simulink model "HexWaRo_StAc_WS_MD"  (Simulink 8.0)
settings: Solver=ode3  StartTime=0.0  StopTime=SimTime  FixedStep=0.02  RelTol=1e-3
values from neighbouring files (symbols this model uses):
  Dgain = -50    [ContinLearn.m]    (also in LearnEvaluation.m; StAcEval.m)
  Kgain = -1500    [ContinLearn.m]    (also in LearnEvaluation.m; StAcEval.m)
  SimTime = .5    (= 0.5)    [ContinLearn.m]    (also in LearnEvaluation.m; StAcEval.m)
  ThetaB = StDeg(st)    [ContinLearn.m]    (also in LearnEvaluation.m; StAcEval.m)
  ThetaE = StDeg(ac)    [ContinLearn.m]    (also in LearnEvaluation.m; StAcEval.m)
libraries: mblibv1 x86
(part 2 of 2)

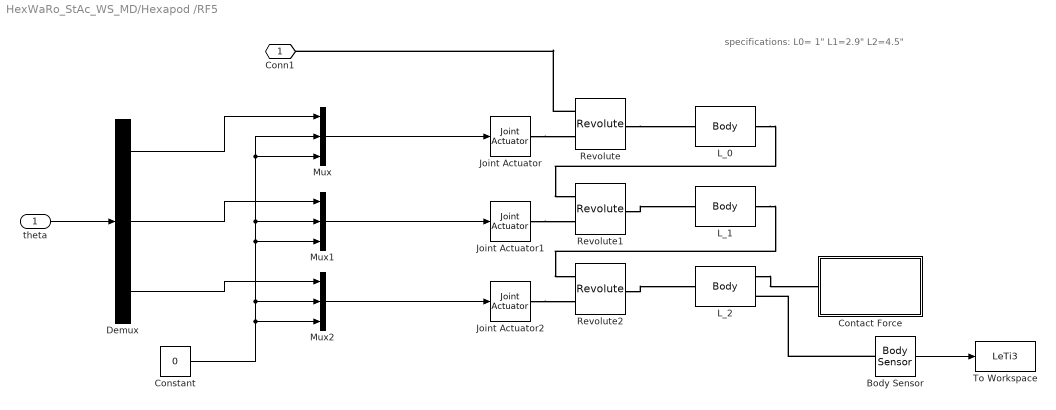
== system HexWaRo_StAc_WS_MD/Hexapod /RF5 ==
  note: specifications:
      | L0= 1"
      | L1=2.9"
      | L2=4.5"
  "theta " : Inport
  Body Sensor : mblibv1/Sensors &  Actuators/Body Sensor  UpdateFromCAD=off  PhysicalDomain=Mechanical  PortType=blob  Muxed=on  Pose=off  Angle=on  AngleUnits=deg  ArcVelocity=off  ArcVelocityUnits=deg/s  ArcAcceleration=off  ArcAccelerationUnits=deg/s^2  CoordPosition=on  CoordPositionUnits=m  Velocity=off  VelocityUnits=m/s  Acceleration=off  AccelerationUnits=m/s^2  Quaternion=on  QuaternionDT=off  QuaternionDDT=off  QuaternionUnits=off  OutputVector=[1]  ActiveIO=on  Width=3  DialogClass=MechanicalSensorBlock  ReferenceFrame=Absolute (World)
  Constant : Constant  Value=0
  Contact Force : Subsystem
  Demux : Demux  Outputs=3
  Joint Actuator : mblibv1/Sensors &  Actuators/Joint Actuator  UpdateFromCAD=off  PhysicalDomain=Mechanical  PortType=blob  ActuationStyle=Motion  AngleUnits=rad  ArcVelocityUnits=rad/s  ArcAccelerationUnits=deg/s^2  CoordPositionUnits=m  VelocityUnits=m/s  AccelerationUnits=m/s^2  ForceUnits=N  TorqueUnits=N*m  ActiveIO=on  Width=3  DialogClass=MechanicalActuatorBlock  Primitive=R1  ReferenceFrame=Absolute (World)
  Joint Actuator1 : mblibv1/Sensors &  Actuators/Joint Actuator  UpdateFromCAD=off  PhysicalDomain=Mechanical  PortType=blob  ActuationStyle=Motion  AngleUnits=rad  ArcVelocityUnits=deg/s  ArcAccelerationUnits=deg/s^2  CoordPositionUnits=m  VelocityUnits=m/s  AccelerationUnits=m/s^2  ForceUnits=N  TorqueUnits=N*m  ActiveIO=on  Width=3  DialogClass=MechanicalActuatorBlock  Primitive=R1  ReferenceFrame=Absolute (World)
  Joint Actuator2 : mblibv1/Sensors &  Actuators/Joint Actuator  UpdateFromCAD=off  PhysicalDomain=Mechanical  PortType=blob  ActuationStyle=Motion  AngleUnits=rad  ArcVelocityUnits=deg/s  ArcAccelerationUnits=deg/s^2  CoordPositionUnits=m  VelocityUnits=m/s  AccelerationUnits=m/s^2  ForceUnits=N  TorqueUnits=N*m  ActiveIO=on  Width=3  DialogClass=MechanicalActuatorBlock  Primitive=R1  ReferenceFrame=Absolute (World)
  L_0 : mblibv1/Bodies/Body  LConnTagsString=CS1  RConnTagsString=CS2  UpdateFromCAD=off  DialogClass=MechanicalBodyBlock  Mass=.1  MassUnits=kg  InertiaUnits=kg*m^2  Inertia=eye(3)  Shape=Cylinder  ShapeDims=[1 1]  ShapeUnits=m  ShapeUse=false  Density=1  DensityUnits=kg/m^3  DensityUse=false  GraphicsMode=MACHINE_DEFAULT  BodyColorSelMode=MACHINE_DEFAULT  BodyColor=[1 0 0]  AttachedToCS=CG  CG=Left$CG$[1.25 0 0]$CS1$CS1$cm$[0 0 0]$Euler X-Y-Z$deg$WORLD$false$none  WorkingFrames=Left$CS1$[0 0 0]$Adjoining$Adjoining$cm$[0 0 0]$Euler X-Y-Z$deg$WORLD$true$none#Right$CS2$[2.5 0 0]$CS1$CS1$cm$[0 0 0]$Euler X-Y-Z$deg$WORLD$true$none  CGPos=[1.25 0 0]  CGRot=[0 0 0]  CS0Pos=[]  CS0Rot=[]  CS1Pos=[0 0 0]  CS1Rot=[0 0 0]  CS2Pos=[2.5 0 0]  CS2Rot=[0 0 0]  CS3Pos=[]  CS3Rot=[]  CS4Pos=[]  CS4Rot=[]  CS5Pos=[]  CS5Rot=[]  CS6Pos=[]  CS6Rot=[]  CS7Pos=[]  CS7Rot=[]  CS8Pos=[]  CS8Rot=[]  CS9Pos=[]  CS9Rot=[]  CS10Pos=[]  CS10Rot=[]  CS11Pos=[]  CS11Rot=[]  CS12Pos=[]  CS12Rot=[]  CS13Pos=[]  CS13Rot=[]  CS14Pos=[]  CS14Rot=[]  CS15Pos=[]  CS15Rot=[]  CS16Pos=[]  CS16Rot=[]  CS17Pos=[]  CS17Rot=[]  CS18Pos=[]  CS18Rot=[]  CS19Pos=[]  CS19Rot=[]  CS20Pos=[]  CS20Rot=[]
  L_1 : mblibv1/Bodies/Body  LConnTagsString=CS1  RConnTagsString=CS2  UpdateFromCAD=off  DialogClass=MechanicalBodyBlock  Mass=.1  MassUnits=kg  InertiaUnits=kg*m^2  Inertia=eye(3)  Shape=Cylinder  ShapeDims=[1 1]  ShapeUnits=m  ShapeUse=false  Density=1  DensityUnits=kg/m^3  DensityUse=false  GraphicsMode=MACHINE_DEFAULT  BodyColorSelMode=MACHINE_DEFAULT  BodyColor=[1 0 0]  AttachedToCS=CG  CG=Left$CG$[3.7 0 0]$CS1$CS1$cm$[0 0 0]$Euler X-Y-Z$deg$WORLD$false$none  WorkingFrames=Left$CS1$[0 0 0]$Adjoining$Adjoining$cm$[0 0 0]$Euler X-Y-Z$deg$WORLD$true$none#Right$CS2$[7.4 0 0]$CS1$CS1$cm$[0 0 0]$Euler X-Y-Z$deg$WORLD$true$none  CGPos=[3.7 0 0]  CGRot=[0 0 0]  CS0Pos=[]  CS0Rot=[]  CS1Pos=[0 0 0]  CS1Rot=[0 0 0]  CS2Pos=[7.4 0 0]  CS2Rot=[0 0 0]  CS3Pos=[]  CS3Rot=[]  CS4Pos=[]  CS4Rot=[]  CS5Pos=[]  CS5Rot=[]  CS6Pos=[]  CS6Rot=[]  CS7Pos=[]  CS7Rot=[]  CS8Pos=[]  CS8Rot=[]  CS9Pos=[]  CS9Rot=[]  CS10Pos=[]  CS10Rot=[]  CS11Pos=[]  CS11Rot=[]  CS12Pos=[]  CS12Rot=[]  CS13Pos=[]  CS13Rot=[]  CS14Pos=[]  CS14Rot=[]  CS15Pos=[]  CS15Rot=[]  CS16Pos=[]  CS16Rot=[]  CS17Pos=[]  CS17Rot=[]  CS18Pos=[]  CS18Rot=[]  CS19Pos=[]  CS19Rot=[]  CS20Pos=[]  CS20Rot=[]
  L_2 : mblibv1/Bodies/Body  LConnTagsString=CS1  RConnTagsString=CS2|CS3  UpdateFromCAD=off  DialogClass=MechanicalBodyBlock  Mass=.1  MassUnits=kg  InertiaUnits=kg*m^2  Inertia=eye(3)  Shape=Cylinder  ShapeDims=[1 1]  ShapeUnits=m  ShapeUse=false  Density=1  DensityUnits=kg/m^3  DensityUse=false  GraphicsMode=MACHINE_DEFAULT  BodyColorSelMode=MACHINE_DEFAULT  BodyColor=[1 0 0]  AttachedToCS=CG  CG=Left$CG$[5.7 0 0]$CS1$CS1$cm$[0 0 0]$Euler X-Y-Z$deg$WORLD$false$none  WorkingFrames=Left$CS1$[0 0 0]$Adjoining$Adjoining$cm$[0 0 0]$Euler X-Y-Z$deg$WORLD$true$none#Right$CS2$[11.4 0 0]$CS1$CS1$cm$[0 0 0]$Euler X-Y-Z$deg$WORLD$true$none#Right$CS3$[11.4 0 0]$CS1$CS1$cm$[0 0 0]$Euler X-Y-Z$deg$WORLD$true$none  CGPos=[5.7 0 0]  CGRot=[0 0 0]  CS0Pos=[]  CS0Rot=[]  CS1Pos=[0 0 0]  CS1Rot=[0 0 0]  CS2Pos=[11.4 0 0]  CS2Rot=[0 0 0]  CS3Pos=[11.4 0 0]  CS3Rot=[0 0 0]  CS4Pos=[]  CS4Rot=[]  CS5Pos=[]  CS5Rot=[]  CS6Pos=[]  CS6Rot=[]  CS7Pos=[]  CS7Rot=[]  CS8Pos=[]  CS8Rot=[]  CS9Pos=[]  CS9Rot=[]  CS10Pos=[]  CS10Rot=[]  CS11Pos=[]  CS11Rot=[]  CS12Pos=[]  CS12Rot=[]  CS13Pos=[]  CS13Rot=[]  CS14Pos=[]  CS14Rot=[]  CS15Pos=[]  CS15Rot=[]  CS16Pos=[]  CS16Rot=[]  CS17Pos=[]  CS17Rot=[]  CS18Pos=[]  CS18Rot=[]  CS19Pos=[]  CS19Rot=[]  CS20Pos=[]  CS20Rot=[]
  Mux : Mux  Inputs=3
  Mux1 : Mux  Inputs=3
  Mux2 : Mux  Inputs=3
  Revolute : mblibv1/Joints/Revolute  LConnTagsString=__newl0|SA1  RConnTagsString=__newr0  UpdateFromCAD=off  NumSAPorts=1  CutJoint=off  MarkAsCut=off  Primitives=prismatic  PrimitiveProps=R1$World$[0 0 1]$revolute  DialogClass=JointBlock  R1Axis=[0 0 1]
  Revolute1 : mblibv1/Joints/Revolute  LConnTagsString=__newl0|SA1  RConnTagsString=__newr0  UpdateFromCAD=off  NumSAPorts=1  CutJoint=off  MarkAsCut=off  Primitives=prismatic  PrimitiveProps=R1$Base$[0 1 0]$revolute  DialogClass=JointBlock  R1Axis=[0 1 0]
  Revolute2 : mblibv1/Joints/Revolute  LConnTagsString=__newl0|SA1  RConnTagsString=__newr0  UpdateFromCAD=off  NumSAPorts=1  CutJoint=off  MarkAsCut=off  Primitives=prismatic  PrimitiveProps=R1$Base$[0 1 0]$revolute  DialogClass=JointBlock  R1Axis=[0 1 0]
  To Workspace : ToWorkspace  VariableName=LeTi3  SampleTime=-1
  Conn1 : PMIOPort  Port=1  Side=Left
  wires:
  "theta "/1 -> Demux/1
  Constant/1 -> Mux2/2, Mux1/3, Mux1/2, Mux/3, Mux/2, Mux2/3
  Demux/3 -> Mux2/1
  Demux/2 -> Mux1/1
  Demux/1 -> Mux/1
  Mux/1 -> Joint Actuator/1
  Mux1/1 -> Joint Actuator1/1
  Mux2/1 -> Joint Actuator2/1
  Body Sensor/1 -> To Workspace/1
  connections:
  Revolute1/RConn1 -- L_1/LConn1
  Revolute2/RConn1 -- L_2/LConn1
  Joint Actuator2/RConn1 -- Revolute2/LConn2
  Joint Actuator/RConn1 -- Revolute/LConn2
  Joint Actuator1/RConn1 -- Revolute1/LConn2
  Revolute/LConn1 -- Conn1/RConn1
  Revolute/RConn1 -- L_0/LConn1
  L_1/RConn1 -- Revolute2/LConn1
  L_0/RConn1 -- Revolute1/LConn1
  L_2/RConn1 -- Contact Force/LConn1
  Body Sensor/LConn1 -- L_2/RConn2

== system HexWaRo_StAc_WS_MD/Hexapod /RF/Contact Force ==
  Body Actuator : mblibv1/Sensors &  Actuators/Body Actuator  UpdateFromCAD=off  PhysicalDomain=Mechanical  PortType=blob  ActuationStyle=Force  AngleUnits=deg  ArcVelocityUnits=deg/s  ArcAccelerationUnits=deg/s^2  CoordPositionUnits=m  VelocityUnits=m/s  AccelerationUnits=m/s^2  ForceUnits=N  TorqueUnits=N-m  ActiveIO=on  Width=3  DialogClass=MechanicalActuatorBlock  ReferenceFrame=Absolute (INERTIAL)  Angle=off  CoordPosition=on  Force=on  Torque=off
  Body Sensor : mblibv1/Sensors &  Actuators/Body Sensor  UpdateFromCAD=off  PhysicalDomain=Mechanical  PortType=blob  Muxed=off  Pose=off  Angle=on  AngleUnits=deg  ArcVelocity=off  ArcVelocityUnits=deg/s  ArcAcceleration=off  ArcAccelerationUnits=deg/s^2  CoordPosition=on  CoordPositionUnits=m  Velocity=on  VelocityUnits=m/s  Acceleration=off  AccelerationUnits=m/s^2  Quaternion=on  QuaternionDT=off  QuaternionDDT=off  QuaternionUnits=off  OutputVector=[ 3 3 ]  ActiveIO=on  Width=6  DialogClass=MechanicalSensorBlock  ReferenceFrame=Absolute (World)
  Force Law : Subsystem
  Mechanical Branching Bar : mblibv1/Utilities/Mechanical Branching Bar  LConnTagsString=_newl0  RConnTagsString=SA0|SA1  UpdateFromCAD=off  DialogClass=MechanicalBranchingBarBlock  NumSAPorts=2
  CG : PMIOPort  Tag=PMCPort  Port=1  Side=Left
  wires:
  Force Law/1(force) -> Body Actuator/1  "Force (N)"
  Body Sensor/2 -> Force Law/2(vel)  "Velocity (m/s)"
  Body Sensor/1 -> Force Law/1(pos)  "Position (m)"
  connections:
  Body Sensor/LConn1 -- Mechanical Branching Bar/RConn1
  Body Actuator/RConn1 -- Mechanical Branching Bar/RConn2
  Mechanical Branching Bar/LConn1 -- CG/RConn1

== system HexWaRo_StAc_WS_MD/Hexapod /RF1/Contact Force ==
  Body Actuator : mblibv1/Sensors &  Actuators/Body Actuator  UpdateFromCAD=off  PhysicalDomain=Mechanical  PortType=blob  ActuationStyle=Force  AngleUnits=deg  ArcVelocityUnits=deg/s  ArcAccelerationUnits=deg/s^2  CoordPositionUnits=m  VelocityUnits=m/s  AccelerationUnits=m/s^2  ForceUnits=N  TorqueUnits=N-m  ActiveIO=on  Width=3  DialogClass=MechanicalActuatorBlock  ReferenceFrame=Absolute (INERTIAL)  Angle=off  CoordPosition=on  Force=on  Torque=off
  Body Sensor : mblibv1/Sensors &  Actuators/Body Sensor  UpdateFromCAD=off  PhysicalDomain=Mechanical  PortType=blob  Muxed=off  Pose=off  Angle=on  AngleUnits=deg  ArcVelocity=off  ArcVelocityUnits=deg/s  ArcAcceleration=off  ArcAccelerationUnits=deg/s^2  CoordPosition=on  CoordPositionUnits=m  Velocity=on  VelocityUnits=m/s  Acceleration=off  AccelerationUnits=m/s^2  Quaternion=on  QuaternionDT=off  QuaternionDDT=off  QuaternionUnits=off  OutputVector=[ 3 3 ]  ActiveIO=on  Width=6  DialogClass=MechanicalSensorBlock  ReferenceFrame=Absolute (World)
  Force Law : Subsystem
  Mechanical Branching Bar : mblibv1/Utilities/Mechanical Branching Bar  LConnTagsString=_newl0  RConnTagsString=SA0|SA1  UpdateFromCAD=off  DialogClass=MechanicalBranchingBarBlock  NumSAPorts=2
  CG : PMIOPort  Tag=PMCPort  Port=1  Side=Left
  wires:
  Body Sensor/1 -> Force Law/1(pos)  "Position (m)"
  Body Sensor/2 -> Force Law/2(vel)  "Velocity (m/s)"
  Force Law/1(force) -> Body Actuator/1  "Force (N)"
  connections:
  Mechanical Branching Bar/LConn1 -- CG/RConn1
  Body Actuator/RConn1 -- Mechanical Branching Bar/RConn2
  Body Sensor/LConn1 -- Mechanical Branching Bar/RConn1

== system HexWaRo_StAc_WS_MD/Hexapod /RF2/Contact Force ==
  Body Actuator : mblibv1/Sensors &  Actuators/Body Actuator  UpdateFromCAD=off  PhysicalDomain=Mechanical  PortType=blob  ActuationStyle=Force  AngleUnits=deg  ArcVelocityUnits=deg/s  ArcAccelerationUnits=deg/s^2  CoordPositionUnits=m  VelocityUnits=m/s  AccelerationUnits=m/s^2  ForceUnits=N  TorqueUnits=N-m  ActiveIO=on  Width=3  DialogClass=MechanicalActuatorBlock  ReferenceFrame=Absolute (INERTIAL)  Angle=off  CoordPosition=on  Force=on  Torque=off
  Body Sensor : mblibv1/Sensors &  Actuators/Body Sensor  UpdateFromCAD=off  PhysicalDomain=Mechanical  PortType=blob  Muxed=off  Pose=off  Angle=on  AngleUnits=deg  ArcVelocity=off  ArcVelocityUnits=deg/s  ArcAcceleration=off  ArcAccelerationUnits=deg/s^2  CoordPosition=on  CoordPositionUnits=m  Velocity=on  VelocityUnits=m/s  Acceleration=off  AccelerationUnits=m/s^2  Quaternion=on  QuaternionDT=off  QuaternionDDT=off  QuaternionUnits=off  OutputVector=[ 3 3 ]  ActiveIO=on  Width=6  DialogClass=MechanicalSensorBlock  ReferenceFrame=Absolute (World)
  Force Law : Subsystem
  Mechanical Branching Bar : mblibv1/Utilities/Mechanical Branching Bar  LConnTagsString=_newl0  RConnTagsString=SA0|SA1  UpdateFromCAD=off  DialogClass=MechanicalBranchingBarBlock  NumSAPorts=2
  CG : PMIOPort  Tag=PMCPort  Port=1  Side=Left
  wires:
  Force Law/1(force) -> Body Actuator/1  "Force (N)"
  Body Sensor/2 -> Force Law/2(vel)  "Velocity (m/s)"
  Body Sensor/1 -> Force Law/1(pos)  "Position (m)"
  connections:
  Body Sensor/LConn1 -- Mechanical Branching Bar/RConn1
  Body Actuator/RConn1 -- Mechanical Branching Bar/RConn2
  Mechanical Branching Bar/LConn1 -- CG/RConn1

== system HexWaRo_StAc_WS_MD/Hexapod /RF3/Contact Force ==
  Body Actuator : mblibv1/Sensors &  Actuators/Body Actuator  UpdateFromCAD=off  PhysicalDomain=Mechanical  PortType=blob  ActuationStyle=Force  AngleUnits=deg  ArcVelocityUnits=deg/s  ArcAccelerationUnits=deg/s^2  CoordPositionUnits=m  VelocityUnits=m/s  AccelerationUnits=m/s^2  ForceUnits=N  TorqueUnits=N-m  ActiveIO=on  Width=3  DialogClass=MechanicalActuatorBlock  ReferenceFrame=Absolute (INERTIAL)  Angle=off  CoordPosition=on  Force=on  Torque=off
  Body Sensor : mblibv1/Sensors &  Actuators/Body Sensor  UpdateFromCAD=off  PhysicalDomain=Mechanical  PortType=blob  Muxed=off  Pose=off  Angle=on  AngleUnits=deg  ArcVelocity=off  ArcVelocityUnits=deg/s  ArcAcceleration=off  ArcAccelerationUnits=deg/s^2  CoordPosition=on  CoordPositionUnits=m  Velocity=on  VelocityUnits=m/s  Acceleration=off  AccelerationUnits=m/s^2  Quaternion=on  QuaternionDT=off  QuaternionDDT=off  QuaternionUnits=off  OutputVector=[ 3 3 ]  ActiveIO=on  Width=6  DialogClass=MechanicalSensorBlock  ReferenceFrame=Absolute (World)
  Force Law : Subsystem
  Mechanical Branching Bar : mblibv1/Utilities/Mechanical Branching Bar  LConnTagsString=_newl0  RConnTagsString=SA0|SA1  UpdateFromCAD=off  DialogClass=MechanicalBranchingBarBlock  NumSAPorts=2
  CG : PMIOPort  Tag=PMCPort  Port=1  Side=Left
  wires:
  Body Sensor/1 -> Force Law/1(pos)  "Position (m)"
  Body Sensor/2 -> Force Law/2(vel)  "Velocity (m/s)"
  Force Law/1(force) -> Body Actuator/1  "Force (N)"
  connections:
  Mechanical Branching Bar/LConn1 -- CG/RConn1
  Body Actuator/RConn1 -- Mechanical Branching Bar/RConn2
  Body Sensor/LConn1 -- Mechanical Branching Bar/RConn1

== system HexWaRo_StAc_WS_MD/Hexapod /RF4/Contact Force ==
  Body Actuator : mblibv1/Sensors &  Actuators/Body Actuator  UpdateFromCAD=off  PhysicalDomain=Mechanical  PortType=blob  ActuationStyle=Force  AngleUnits=deg  ArcVelocityUnits=deg/s  ArcAccelerationUnits=deg/s^2  CoordPositionUnits=m  VelocityUnits=m/s  AccelerationUnits=m/s^2  ForceUnits=N  TorqueUnits=N-m  ActiveIO=on  Width=3  DialogClass=MechanicalActuatorBlock  ReferenceFrame=Absolute (INERTIAL)  Angle=off  CoordPosition=on  Force=on  Torque=off
  Body Sensor : mblibv1/Sensors &  Actuators/Body Sensor  UpdateFromCAD=off  PhysicalDomain=Mechanical  PortType=blob  Muxed=off  Pose=off  Angle=on  AngleUnits=deg  ArcVelocity=off  ArcVelocityUnits=deg/s  ArcAcceleration=off  ArcAccelerationUnits=deg/s^2  CoordPosition=on  CoordPositionUnits=m  Velocity=on  VelocityUnits=m/s  Acceleration=off  AccelerationUnits=m/s^2  Quaternion=on  QuaternionDT=off  QuaternionDDT=off  QuaternionUnits=off  OutputVector=[ 3 3 ]  ActiveIO=on  Width=6  DialogClass=MechanicalSensorBlock  ReferenceFrame=Absolute (World)
  Force Law : Subsystem
  Mechanical Branching Bar : mblibv1/Utilities/Mechanical Branching Bar  LConnTagsString=_newl0  RConnTagsString=SA0|SA1  UpdateFromCAD=off  DialogClass=MechanicalBranchingBarBlock  NumSAPorts=2
  CG : PMIOPort  Tag=PMCPort  Port=1  Side=Left
  wires:
  Force Law/1(force) -> Body Actuator/1  "Force (N)"
  Body Sensor/2 -> Force Law/2(vel)  "Velocity (m/s)"
  Body Sensor/1 -> Force Law/1(pos)  "Position (m)"
  connections:
  Body Sensor/LConn1 -- Mechanical Branching Bar/RConn1
  Body Actuator/RConn1 -- Mechanical Branching Bar/RConn2
  Mechanical Branching Bar/LConn1 -- CG/RConn1

== system HexWaRo_StAc_WS_MD/Hexapod /RF5/Contact Force ==
  Body Actuator : mblibv1/Sensors &  Actuators/Body Actuator  UpdateFromCAD=off  PhysicalDomain=Mechanical  PortType=blob  ActuationStyle=Force  AngleUnits=deg  ArcVelocityUnits=deg/s  ArcAccelerationUnits=deg/s^2  CoordPositionUnits=m  VelocityUnits=m/s  AccelerationUnits=m/s^2  ForceUnits=N  TorqueUnits=N-m  ActiveIO=on  Width=3  DialogClass=MechanicalActuatorBlock  ReferenceFrame=Absolute (INERTIAL)  Angle=off  CoordPosition=on  Force=on  Torque=off
  Body Sensor : mblibv1/Sensors &  Actuators/Body Sensor  UpdateFromCAD=off  PhysicalDomain=Mechanical  PortType=blob  Muxed=off  Pose=off  Angle=on  AngleUnits=deg  ArcVelocity=off  ArcVelocityUnits=deg/s  ArcAcceleration=off  ArcAccelerationUnits=deg/s^2  CoordPosition=on  CoordPositionUnits=m  Velocity=on  VelocityUnits=m/s  Acceleration=off  AccelerationUnits=m/s^2  Quaternion=on  QuaternionDT=off  QuaternionDDT=off  QuaternionUnits=off  OutputVector=[ 3 3 ]  ActiveIO=on  Width=6  DialogClass=MechanicalSensorBlock  ReferenceFrame=Absolute (World)
  Force Law : Subsystem
  Mechanical Branching Bar : mblibv1/Utilities/Mechanical Branching Bar  LConnTagsString=_newl0  RConnTagsString=SA0|SA1  UpdateFromCAD=off  DialogClass=MechanicalBranchingBarBlock  NumSAPorts=2
  CG : PMIOPort  Tag=PMCPort  Port=1  Side=Left
  wires:
  Body Sensor/1 -> Force Law/1(pos)  "Position (m)"
  Body Sensor/2 -> Force Law/2(vel)  "Velocity (m/s)"
  Force Law/1(force) -> Body Actuator/1  "Force (N)"
  connections:
  Mechanical Branching Bar/LConn1 -- CG/RConn1
  Body Actuator/RConn1 -- Mechanical Branching Bar/RConn2
  Body Sensor/LConn1 -- Mechanical Branching Bar/RConn1

== system HexWaRo_StAc_WS_MD/Hexapod /RF/Contact Force/Force Law ==
  pos : Inport
  vel : Inport  Port=2
  Constant : Constant  Value=0
  If : If  IfExpression=u1 < 0
  Merge : Merge  InitialOutput=0  InputPortOffsets=0
  Penalty Force : Subsystem  TreatAsAtomicUnit=on
  Selector : Selector  InputPortWidth=3  IndexOptions=Index vector (dialog)  Indices=[3]  OutputSizes=1
  Sum : Sum  Inputs=-+|  SaturateOnIntegerOverflow=on
  Zero Force : Subsystem  TreatAsAtomicUnit=on
  force : Outport
  wires:
  Selector/1 -> If/1
  If/1 -> Penalty Force/Action
  Merge/1 -> force/1
  Zero Force/1(force) -> Merge/2
  Penalty Force/1(force) -> Merge/1
  If/2 -> Zero Force/Action
  vel/1 -> Penalty Force/2(vel)
  Constant/1 -> Sum/1
  Sum/1 -> Penalty Force/1(pen), Selector/1
  pos/1 -> Sum/2

== system HexWaRo_StAc_WS_MD/Hexapod /RF1/Contact Force/Force Law ==
  pos : Inport
  vel : Inport  Port=2
  Constant : Constant  Value=0
  If : If  IfExpression=u1 < 0
  Merge : Merge  InitialOutput=0  InputPortOffsets=0
  Penalty Force : Subsystem  TreatAsAtomicUnit=on
  Selector : Selector  InputPortWidth=3  IndexOptions=Index vector (dialog)  Indices=[3]  OutputSizes=1
  Sum : Sum  Inputs=-+|  SaturateOnIntegerOverflow=on
  Zero Force : Subsystem  TreatAsAtomicUnit=on
  force : Outport
  wires:
  pos/1 -> Sum/2
  Sum/1 -> Selector/1, Penalty Force/1(pen)
  Constant/1 -> Sum/1
  vel/1 -> Penalty Force/2(vel)
  If/2 -> Zero Force/Action
  Penalty Force/1(force) -> Merge/1
  Zero Force/1(force) -> Merge/2
  Merge/1 -> force/1
  If/1 -> Penalty Force/Action
  Selector/1 -> If/1

== system HexWaRo_StAc_WS_MD/Hexapod /RF2/Contact Force/Force Law ==
  pos : Inport
  vel : Inport  Port=2
  Constant : Constant  Value=0
  If : If  IfExpression=u1 < 0
  Merge : Merge  InitialOutput=0  InputPortOffsets=0
  Penalty Force : Subsystem  TreatAsAtomicUnit=on
  Selector : Selector  InputPortWidth=3  IndexOptions=Index vector (dialog)  Indices=[3]  OutputSizes=1
  Sum : Sum  Inputs=-+|  SaturateOnIntegerOverflow=on
  Zero Force : Subsystem  TreatAsAtomicUnit=on
  force : Outport
  wires:
  Selector/1 -> If/1
  If/1 -> Penalty Force/Action
  Merge/1 -> force/1
  Zero Force/1(force) -> Merge/2
  Penalty Force/1(force) -> Merge/1
  If/2 -> Zero Force/Action
  vel/1 -> Penalty Force/2(vel)
  Constant/1 -> Sum/1
  Sum/1 -> Penalty Force/1(pen), Selector/1
  pos/1 -> Sum/2

== system HexWaRo_StAc_WS_MD/Hexapod /RF3/Contact Force/Force Law ==
  pos : Inport
  vel : Inport  Port=2
  Constant : Constant  Value=0
  If : If  IfExpression=u1 < 0
  Merge : Merge  InitialOutput=0  InputPortOffsets=0
  Penalty Force : Subsystem  TreatAsAtomicUnit=on
  Selector : Selector  InputPortWidth=3  IndexOptions=Index vector (dialog)  Indices=[3]  OutputSizes=1
  Sum : Sum  Inputs=-+|  SaturateOnIntegerOverflow=on
  Zero Force : Subsystem  TreatAsAtomicUnit=on
  force : Outport
  wires:
  pos/1 -> Sum/2
  Sum/1 -> Selector/1, Penalty Force/1(pen)
  Constant/1 -> Sum/1
  vel/1 -> Penalty Force/2(vel)
  If/2 -> Zero Force/Action
  Penalty Force/1(force) -> Merge/1
  Zero Force/1(force) -> Merge/2
  Merge/1 -> force/1
  If/1 -> Penalty Force/Action
  Selector/1 -> If/1

== system HexWaRo_StAc_WS_MD/Hexapod /RF4/Contact Force/Force Law ==
  pos : Inport
  vel : Inport  Port=2
  Constant : Constant  Value=0
  If : If  IfExpression=u1 < 0
  Merge : Merge  InitialOutput=0  InputPortOffsets=0
  Penalty Force : Subsystem  TreatAsAtomicUnit=on
  Selector : Selector  InputPortWidth=3  IndexOptions=Index vector (dialog)  Indices=[3]  OutputSizes=1
  Sum : Sum  Inputs=-+|  SaturateOnIntegerOverflow=on
  Zero Force : Subsystem  TreatAsAtomicUnit=on
  force : Outport
  wires:
  Selector/1 -> If/1
  If/1 -> Penalty Force/Action
  Merge/1 -> force/1
  Zero Force/1(force) -> Merge/2
  Penalty Force/1(force) -> Merge/1
  If/2 -> Zero Force/Action
  vel/1 -> Penalty Force/2(vel)
  Constant/1 -> Sum/1
  Sum/1 -> Penalty Force/1(pen), Selector/1
  pos/1 -> Sum/2

== system HexWaRo_StAc_WS_MD/Hexapod /RF5/Contact Force/Force Law ==
  pos : Inport
  vel : Inport  Port=2
  Constant : Constant  Value=0
  If : If  IfExpression=u1 < 0
  Merge : Merge  InitialOutput=0  InputPortOffsets=0
  Penalty Force : Subsystem  TreatAsAtomicUnit=on
  Selector : Selector  InputPortWidth=3  IndexOptions=Index vector (dialog)  Indices=[3]  OutputSizes=1
  Sum : Sum  Inputs=-+|  SaturateOnIntegerOverflow=on
  Zero Force : Subsystem  TreatAsAtomicUnit=on
  force : Outport
  wires:
  pos/1 -> Sum/2
  Sum/1 -> Selector/1, Penalty Force/1(pen)
  Constant/1 -> Sum/1
  vel/1 -> Penalty Force/2(vel)
  If/2 -> Zero Force/Action
  Penalty Force/1(force) -> Merge/1
  Zero Force/1(force) -> Merge/2
  Merge/1 -> force/1
  If/1 -> Penalty Force/Action
  Selector/1 -> If/1

== system HexWaRo_StAc_WS_MD/Hexapod /RF/Contact Force/Force Law/Penalty Force ==
  pen : Inport
  vel : Inport  Port=2
  Action Port : ActionPort  ActionType=then
  Gain : Gain  Gain=[0 0 0;0 0 0;0 0 Kgain]  Multiplication=Matrix(K*u)  SaturateOnIntegerOverflow=on  OutDataTypeStr=Inherit: Same as input  ParamDataTypeStr=Inherit: Same as input
  Gain1 : Gain  Gain=[0 0 0;0 0 0;0 0 Dgain]  Multiplication=Matrix(K*u)  SaturateOnIntegerOverflow=on  OutDataTypeStr=Inherit: Same as input  ParamDataTypeStr=Inherit: Same as input
  Saturation : Saturate  UpperLimit=inf  LowerLimit=0
  Sum : Sum  Inputs=|++  SaturateOnIntegerOverflow=on
  force : Outport  InitialOutput=0
  wires:
  Saturation/1 -> force/1
  vel/1 -> Gain1/1
  Gain1/1 -> Sum/2
  Sum/1 -> Saturation/1
  Gain/1 -> Sum/1
  pen/1 -> Gain/1

== system HexWaRo_StAc_WS_MD/Hexapod /RF/Contact Force/Force Law/Zero Force ==
  Action Port : ActionPort  ActionType=else
  Zero Force : Constant  Value=[0;0;0]
  force : Outport  InitialOutput=0
  wires:
  Zero Force/1 -> force/1

== system HexWaRo_StAc_WS_MD/Hexapod /RF1/Contact Force/Force Law/Penalty Force ==
  pen : Inport
  vel : Inport  Port=2
  Action Port : ActionPort  ActionType=then
  Gain : Gain  Gain=[0 0 0;0 0 0;0 0 Kgain]  Multiplication=Matrix(K*u)  SaturateOnIntegerOverflow=on  OutDataTypeStr=Inherit: Same as input  ParamDataTypeStr=Inherit: Same as input
  Gain1 : Gain  Gain=[0 0 0;0 0 0;0 0 Dgain]  Multiplication=Matrix(K*u)  SaturateOnIntegerOverflow=on  OutDataTypeStr=Inherit: Same as input  ParamDataTypeStr=Inherit: Same as input
  Saturation : Saturate  UpperLimit=inf  LowerLimit=0
  Sum : Sum  Inputs=|++  SaturateOnIntegerOverflow=on
  force : Outport  InitialOutput=0
  wires:
  pen/1 -> Gain/1
  Gain/1 -> Sum/1
  Sum/1 -> Saturation/1
  Gain1/1 -> Sum/2
  vel/1 -> Gain1/1
  Saturation/1 -> force/1

== system HexWaRo_StAc_WS_MD/Hexapod /RF1/Contact Force/Force Law/Zero Force ==
  Action Port : ActionPort  ActionType=else
  Zero Force : Constant  Value=[0;0;0]
  force : Outport  InitialOutput=0
  wires:
  Zero Force/1 -> force/1

== system HexWaRo_StAc_WS_MD/Hexapod /RF2/Contact Force/Force Law/Penalty Force ==
  pen : Inport
  vel : Inport  Port=2
  Action Port : ActionPort  ActionType=then
  Gain : Gain  Gain=[0 0 0;0 0 0;0 0 -Kgain]  Multiplication=Matrix(K*u)  SaturateOnIntegerOverflow=on  OutDataTypeStr=Inherit: Same as input  ParamDataTypeStr=Inherit: Same as input
  Gain1 : Gain  Gain=[0 0 0;0 0 0;0 0 Dgain]  Multiplication=Matrix(K*u)  SaturateOnIntegerOverflow=on  OutDataTypeStr=Inherit: Same as input  ParamDataTypeStr=Inherit: Same as input
  Saturation : Saturate  UpperLimit=inf  LowerLimit=0
  Sum : Sum  Inputs=|++  SaturateOnIntegerOverflow=on
  force : Outport  InitialOutput=0
  wires:
  Saturation/1 -> force/1
  vel/1 -> Gain1/1
  Gain1/1 -> Sum/2
  Sum/1 -> Saturation/1
  Gain/1 -> Sum/1
  pen/1 -> Gain/1

== system HexWaRo_StAc_WS_MD/Hexapod /RF2/Contact Force/Force Law/Zero Force ==
  Action Port : ActionPort  ActionType=else
  Zero Force : Constant  Value=[0;0;0]
  force : Outport  InitialOutput=0
  wires:
  Zero Force/1 -> force/1

== system HexWaRo_StAc_WS_MD/Hexapod /RF3/Contact Force/Force Law/Penalty Force ==
  pen : Inport
  vel : Inport  Port=2
  Action Port : ActionPort  ActionType=then
  Gain : Gain  Gain=[0 0 0;0 0 0;0 0 Kgain]  Multiplication=Matrix(K*u)  SaturateOnIntegerOverflow=on  OutDataTypeStr=Inherit: Same as input  ParamDataTypeStr=Inherit: Same as input
  Gain1 : Gain  Gain=[0 0 0;0 0 0;0 0 Dgain]  Multiplication=Matrix(K*u)  SaturateOnIntegerOverflow=on  OutDataTypeStr=Inherit: Same as input  ParamDataTypeStr=Inherit: Same as input
  Saturation : Saturate  UpperLimit=inf  LowerLimit=0
  Sum : Sum  Inputs=|++  SaturateOnIntegerOverflow=on
  force : Outport  InitialOutput=0
  wires:
  pen/1 -> Gain/1
  Gain/1 -> Sum/1
  Sum/1 -> Saturation/1
  Gain1/1 -> Sum/2
  vel/1 -> Gain1/1
  Saturation/1 -> force/1

== system HexWaRo_StAc_WS_MD/Hexapod /RF3/Contact Force/Force Law/Zero Force ==
  Action Port : ActionPort  ActionType=else
  Zero Force : Constant  Value=[0;0;0]
  force : Outport  InitialOutput=0
  wires:
  Zero Force/1 -> force/1

== system HexWaRo_StAc_WS_MD/Hexapod /RF4/Contact Force/Force Law/Penalty Force ==
  pen : Inport
  vel : Inport  Port=2
  Action Port : ActionPort  ActionType=then
  Gain : Gain  Gain=[0 0 0;0 0 0;0 0 Kgain]  Multiplication=Matrix(K*u)  SaturateOnIntegerOverflow=on  OutDataTypeStr=Inherit: Same as input  ParamDataTypeStr=Inherit: Same as input
  Gain1 : Gain  Gain=[0 0 0;0 0 0;0 0 Dgain]  Multiplication=Matrix(K*u)  SaturateOnIntegerOverflow=on  OutDataTypeStr=Inherit: Same as input  ParamDataTypeStr=Inherit: Same as input
  Saturation : Saturate  UpperLimit=inf  LowerLimit=0
  Sum : Sum  Inputs=|++  SaturateOnIntegerOverflow=on
  force : Outport  InitialOutput=0
  wires:
  Saturation/1 -> force/1
  vel/1 -> Gain1/1
  Gain1/1 -> Sum/2
  Sum/1 -> Saturation/1
  Gain/1 -> Sum/1
  pen/1 -> Gain/1

== system HexWaRo_StAc_WS_MD/Hexapod /RF4/Contact Force/Force Law/Zero Force ==
  Action Port : ActionPort  ActionType=else
  Zero Force : Constant  Value=[0;0;0]
  force : Outport  InitialOutput=0
  wires:
  Zero Force/1 -> force/1

== system HexWaRo_StAc_WS_MD/Hexapod /RF5/Contact Force/Force Law/Penalty Force ==
  pen : Inport
  vel : Inport  Port=2
  Action Port : ActionPort  ActionType=then
  Gain : Gain  Gain=[0 0 0;0 0 0;0 0 Kgain]  Multiplication=Matrix(K*u)  SaturateOnIntegerOverflow=on  OutDataTypeStr=Inherit: Same as input  ParamDataTypeStr=Inherit: Same as input
  Gain1 : Gain  Gain=[0 0 0;0 0 0;0 0 Dgain]  Multiplication=Matrix(K*u)  SaturateOnIntegerOverflow=on  OutDataTypeStr=Inherit: Same as input  ParamDataTypeStr=Inherit: Same as input
  Saturation : Saturate  UpperLimit=inf  LowerLimit=0
  Sum : Sum  Inputs=|++  SaturateOnIntegerOverflow=on
  force : Outport  InitialOutput=0
  wires:
  pen/1 -> Gain/1
  Gain/1 -> Sum/1
  Sum/1 -> Saturation/1
  Gain1/1 -> Sum/2
  vel/1 -> Gain1/1
  Saturation/1 -> force/1

== system HexWaRo_StAc_WS_MD/Hexapod /RF5/Contact Force/Force Law/Zero Force ==
  Action Port : ActionPort  ActionType=else
  Zero Force : Constant  Value=[0;0;0]
  force : Outport  InitialOutput=0
  wires:
  Zero Force/1 -> force/1
